simulink model "TP3_simu_realim_obs_ci_continuo"  (R2023b)
settings: Solver=VariableStepAuto  StartTime=0.0  StopTime=6  RelTol=1e-3
values from neighbouring files (symbols this model uses):
  A = sysc .A    [Prueba_Control.m]
  B = sysc .B    [Prueba_Control.m]
  C = sysc .C    [Prueba_Control.m]
  D = sysc .D    [Prueba_Control.m]
  K = place(A ,B ,poles_ctrl)    [Prueba_Control_CI.m]    (also in control3.m = place(A,B,poles_ctrl))
  Ki = Kdi(end)    [Prueba_Control_CI.m]
  L = place(A' , C', poles_obs )'    [Prueba_Control_CI.m]    (also in control3.m = place(A', C', poles_obs)')
  ue = 0    [Prueba_Control_CI.m]    (also in control3.m)
  x1e = 0    [Prueba_Control_CI.m]    (also in control3.m)
  x2e = 0    [Prueba_Control_CI.m]    (also in control3.m)
  x3e = 0    [Prueba_Control_CI.m]    (also in control3.m)
  x4e = 0    [Prueba_Control_CI.m]    (also in control3.m)
  xeq = [x1e;x2e;x3e;x4e]    [Prueba_Control_CI.m]    (also in control3.m)
  ye = x3e    (= 0)    [Prueba_Control_CI.m]    (also in control3.m)
libraries: cstblocks x1
settings Model: Creator=manuh  LastModifiedBy=ApoloXVIII

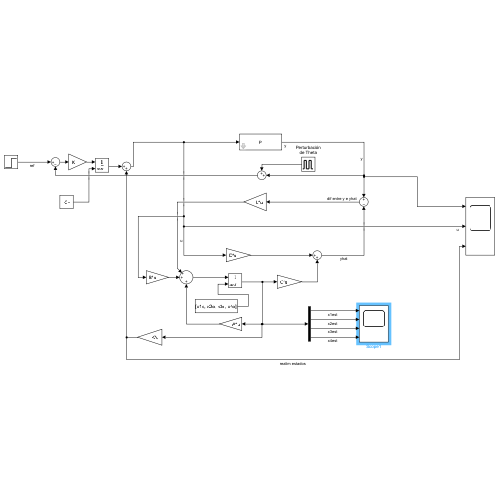
[thumbnail: Simulink's stored preview of the top-level diagram]
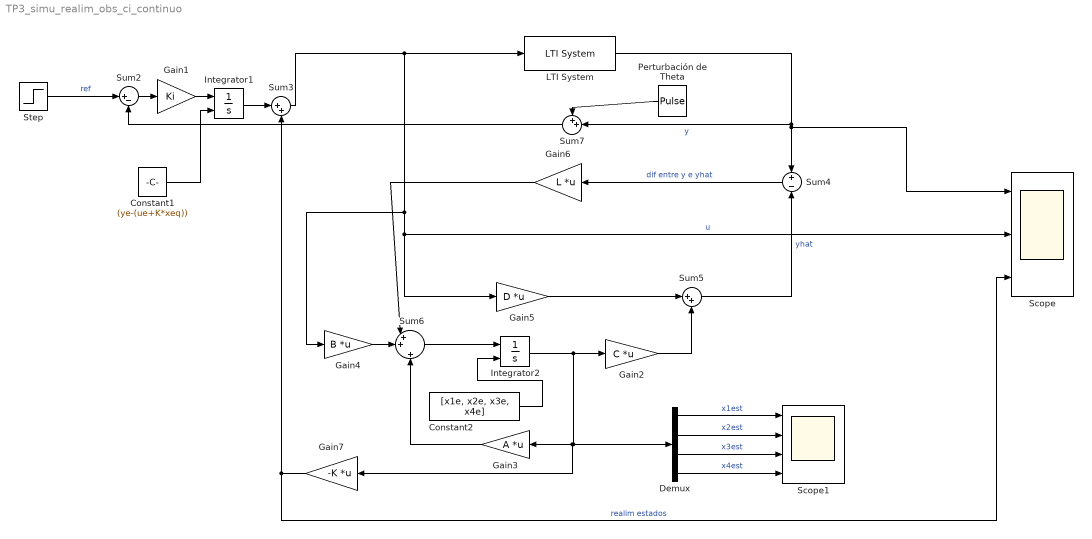
== system TP3_simu_realim_obs_ci_continuo ==
  Constant1 : Constant  Value=(ye-(ue+K*xeq))
  Constant2 : Constant  Value=[x1e, x2e, x3e, x4e]
  Demux : Demux
  Gain1 : Gain  Gain=Ki
  Gain2 : Gain  Gain=C  Multiplication=Matrix(K*u)
  Gain3 : Gain  Gain=A  Multiplication=Matrix(K*u)
  Gain4 : Gain  Gain=B  Multiplication=Matrix(K*u)
  Gain5 : Gain  Gain=D  Multiplication=Matrix(K*u)
  Gain6 : Gain  Gain=L  Multiplication=Matrix(K*u)
  Gain7 : Gain  Gain=-K  Multiplication=Matrix(K*u)
  Integrator1 : Integrator  InitialConditionSource=external
  Integrator2 : Integrator  InitialConditionSource=external
  LTI System : cstblocks/LTI System  sys=P  IC=[]  PadeOrder=0
  Perturbación de Theta : DiscretePulseGenerator  PulseType=Time based  Amplitude=-30  Period=12  PulseWidth=0.3  PhaseDelay=2
  Scope : Scope  NumInputPorts=3
  Scope1 : Scope  NumInputPorts=4
  Step : Step  Time=0  After=0  SampleTime=0
  Sum2 : Sum  Inputs=|+-
  Sum3 : Sum  Inputs=|++
  Sum4 : Sum  Inputs=+|-
  Sum5 : Sum  Inputs=|++
  Sum6 : Sum  Inputs=|++|+
  Sum7 : Sum  Inputs=++|
  wires:
  Step/1 -> Sum2/1  "ref"
  Sum2/1 -> Gain1/1
  Gain1/1 -> Integrator1/1
  Integrator1/1 -> Sum3/1
  Constant1/1 -> Integrator1/2
  Sum3/1 -> Gain5/1, Scope/2, Gain4/1, LTI System/1  "u"
  Sum4/1 -> Gain6/1  "dif entre y e yhat"
  LTI System/1 -> Sum4/1, Scope/1, Sum7/2  "y"
  Gain5/1 -> Sum5/1
  Sum5/1 -> Sum4/2  "yhat"
  Gain2/1 -> Sum5/2
  Integrator2/1 -> Gain7/1, Gain3/1, Demux/1, Gain2/1
  Gain3/1 -> Sum6/3
  Sum6/1 -> Integrator2/1
  Gain4/1 -> Sum6/2
  Gain6/1 -> Sum6/1
  Constant2/1 -> Integrator2/2
  Gain7/1 -> Sum3/2, Scope/3  "realim estados"
  Demux/1 -> Scope1/1  "x1est"
  Demux/2 -> Scope1/2  "x2est"
  Demux/3 -> Scope1/3  "x3est"
  Demux/4 -> Scope1/4  "x4est"
  Perturbación de Theta/1 -> Sum7/1
  Sum7/1 -> Sum2/2
